simulink model "high_pass"  (R2024b)
settings: Solver=VariableStepAuto  StartTime=0.0  StopTime=10.0  RelTol=1e-3
libraries: dspsrcs4 x1
settings Model: Creator=woutlyen  LastModifiedBy=woutlyen

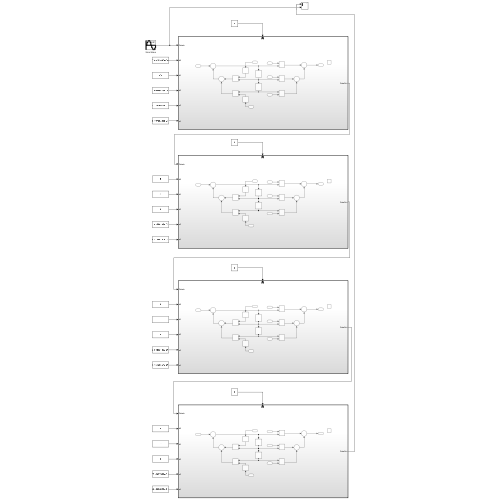
[thumbnail: Simulink's stored preview of the top-level diagram]
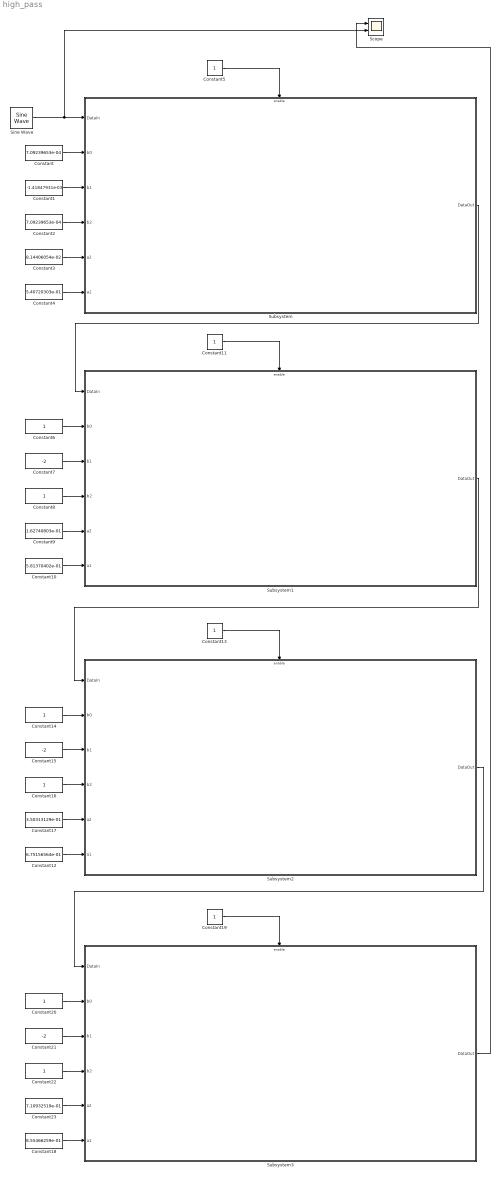
== system high_pass ==
  Constant : Constant  Value=7.09239653e-04  OutDataTypeStr=fixdt(1,27,23)
  Constant1 : Constant  Value=-1.41847931e-03  OutDataTypeStr=fixdt(1,27,23)
  Constant10 : Constant  Value=5.81370402e-01  OutDataTypeStr=fixdt(1,27,23)
  Constant{5,11,13,19} (4 alike) : Constant  OutDataTypeStr=boolean
  Constant12 : Constant  Value=6.75156564e-01  OutDataTypeStr=fixdt(1,27,23)
  Constant{6,8,14,16,20,22} (6 alike) : Constant  OutDataTypeStr=fixdt(1,27,23)
  Constant15 : Constant  Value=-2  OutDataTypeStr=fixdt(1,27,23)
  Constant17 : Constant  Value=3.50313129e-01  OutDataTypeStr=fixdt(1,27,23)
  Constant18 : Constant  Value=8.55466259e-01  OutDataTypeStr=fixdt(1,27,23)
  Constant2 : Constant  Value=7.09239653e-04  OutDataTypeStr=fixdt(1,27,23)
  Constant21 : Constant  Value=-2  OutDataTypeStr=fixdt(1,27,23)
  Constant23 : Constant  Value=7.10932519e-01  OutDataTypeStr=fixdt(1,27,23)
  Constant3 : Constant  Value=8.14406054e-02  OutDataTypeStr=fixdt(1,27,23)
  Constant4 : Constant  Value=5.40720303e-01  OutDataTypeStr=fixdt(1,27,23)
  Constant7 : Constant  Value=-2  OutDataTypeStr=fixdt(1,27,23)
  Constant9 : Constant  Value=1.62740803e-01  OutDataTypeStr=fixdt(1,27,23)
  Scope : Scope  NumInputPorts=2
  Sine Wave : dspsrcs4/Sine Wave  Amplitude=0.6  Frequency=16000  Phase=0  SampleMode=Discrete  OutComplex=Real  CompMethod=Table lookup  TableSize=Speed  SampleTime=1/48000  SamplesPerFrame=1  ResetState=Restart at time zero  OutputFrames=off  dataType=Fixed-point  wordLen=24  udDataType=sfix(16)  fracBitsMode=User-defined  numFracBits=23  OutDataTypeStr=fixdt(1,24,23)  LastOutDataTypeStr=fixdt(1,24,23)
  Subsystem : Subsystem
  Subsystem1 : Subsystem
  Subsystem2 : Subsystem
  Subsystem3 : Subsystem
  wires:
  Constant17/1 -> Subsystem2/5(a2)
  Constant19/1 -> Subsystem3/Enable
  Constant12/1 -> Subsystem2/6(a1)
  Subsystem1/1(DataOut) -> Subsystem2/1(DataIn)
  Constant5/1 -> Subsystem/Enable
  Constant20/1 -> Subsystem3/2(b0)
  Subsystem3/1(DataOut) -> Scope/1
  Constant4/1 -> Subsystem/6(a1)
  Constant18/1 -> Subsystem3/6(a1)
  Subsystem2/1(DataOut) -> Subsystem3/1(DataIn)
  Constant7/1 -> Subsystem1/3(b1)
  Constant13/1 -> Subsystem2/Enable
  Constant/1 -> Subsystem/2(b0)
  Constant22/1 -> Subsystem3/4(b2)
  Constant9/1 -> Subsystem1/5(a2)
  Constant11/1 -> Subsystem1/Enable
  Constant8/1 -> Subsystem1/4(b2)
  Constant1/1 -> Subsystem/3(b1)
  Constant6/1 -> Subsystem1/2(b0)
  Sine Wave/1 -> Scope/2, Subsystem/1(DataIn)
  Constant14/1 -> Subsystem2/2(b0)
  Constant3/1 -> Subsystem/5(a2)
  Constant2/1 -> Subsystem/4(b2)
  Constant10/1 -> Subsystem1/6(a1)
  Subsystem/1(DataOut) -> Subsystem1/1(DataIn)
  Constant15/1 -> Subsystem2/3(b1)
  Constant16/1 -> Subsystem2/4(b2)
  Constant23/1 -> Subsystem3/5(a2)
  Constant21/1 -> Subsystem3/3(b1)

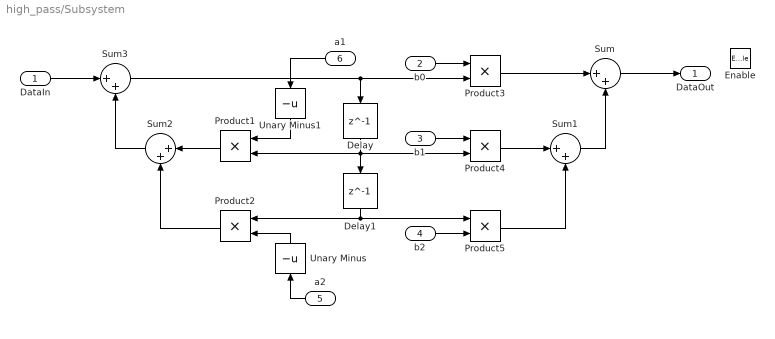
== system high_pass/Subsystem ==
  DataIn : Inport
  b0 : Inport  Port=2
  b1 : Inport  Port=3
  b2 : Inport  Port=4
  a2 : Inport  Port=5
  a1 : Inport  Port=6
  Enable : EnablePort
  Delay : Delay  DelayLength=1  InitialCondition=0
  Delay1 : Delay  DelayLength=1  InitialCondition=0
  Product{1..5} (5 alike) : Product  OutDataTypeStr=fixdt(1,27,23)
  Sum{,1..3} (4 alike) : Sum  Inputs=|++
  Unary Minus : UnaryMinus
  Unary Minus1 : UnaryMinus
  DataOut : Outport  VectorParamsAs1DForOutWhenUnconnected=off
  wires:
  Product4/1 -> Sum1/1
  b1/1 -> Product4/1
  Sum/1 -> DataOut/1
  Sum1/1 -> Sum/2
  b2/1 -> Product5/2
  a2/1 -> Unary Minus/1
  Delay1/1 -> Product2/1, Product5/1
  DataIn/1 -> Sum3/1
  Product2/1 -> Sum2/2
  Sum3/1 -> Delay/1, Product3/2
  Product1/1 -> Sum2/1
  Unary Minus1/1 -> Product1/1
  Sum2/1 -> Sum3/2
  Delay/1 -> Product4/2, Product1/2, Delay1/1
  Product3/1 -> Sum/1
  Unary Minus/1 -> Product2/2
  b0/1 -> Product3/1
  Product5/1 -> Sum1/2
  a1/1 -> Unary Minus1/1

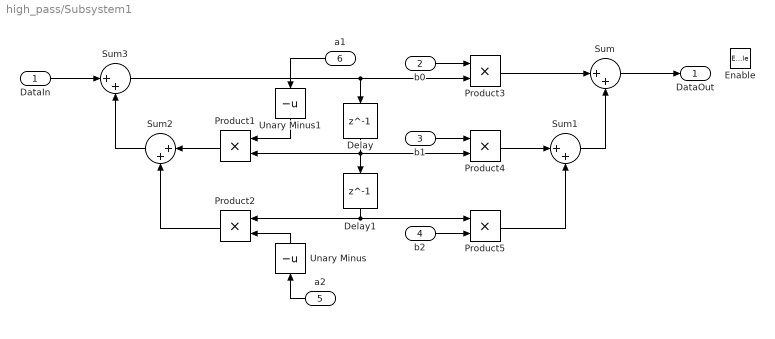
== system high_pass/Subsystem1 ==
  DataIn : Inport
  b0 : Inport  Port=2
  b1 : Inport  Port=3
  b2 : Inport  Port=4
  a2 : Inport  Port=5
  a1 : Inport  Port=6
  Enable : EnablePort
  Delay : Delay  DelayLength=1  InitialCondition=0
  Delay1 : Delay  DelayLength=1  InitialCondition=0
  Product{1..5} (5 alike) : Product  OutDataTypeStr=fixdt(1,27,23)
  Sum{,1..3} (4 alike) : Sum  Inputs=|++
  Unary Minus : UnaryMinus
  Unary Minus1 : UnaryMinus
  DataOut : Outport  VectorParamsAs1DForOutWhenUnconnected=off
  wires:
  Product4/1 -> Sum1/1
  b1/1 -> Product4/1
  Sum/1 -> DataOut/1
  Sum1/1 -> Sum/2
  b2/1 -> Product5/2
  a2/1 -> Unary Minus/1
  Delay1/1 -> Product2/1, Product5/1
  DataIn/1 -> Sum3/1
  Product2/1 -> Sum2/2
  Sum3/1 -> Delay/1, Product3/2
  Product1/1 -> Sum2/1
  Unary Minus1/1 -> Product1/1
  Sum2/1 -> Sum3/2
  Delay/1 -> Product4/2, Product1/2, Delay1/1
  Product3/1 -> Sum/1
  Unary Minus/1 -> Product2/2
  b0/1 -> Product3/1
  Product5/1 -> Sum1/2
  a1/1 -> Unary Minus1/1

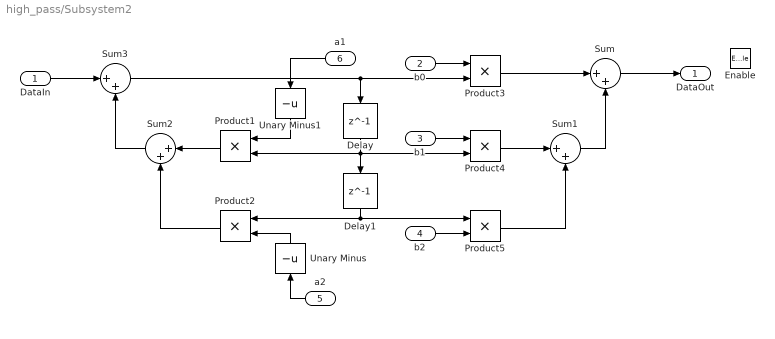
== system high_pass/Subsystem2 ==
  DataIn : Inport
  b0 : Inport  Port=2
  b1 : Inport  Port=3
  b2 : Inport  Port=4
  a2 : Inport  Port=5
  a1 : Inport  Port=6
  Enable : EnablePort
  Delay : Delay  DelayLength=1  InitialCondition=0
  Delay1 : Delay  DelayLength=1  InitialCondition=0
  Product{1..5} (5 alike) : Product  OutDataTypeStr=fixdt(1,27,23)
  Sum{,1..3} (4 alike) : Sum  Inputs=|++
  Unary Minus : UnaryMinus
  Unary Minus1 : UnaryMinus
  DataOut : Outport  VectorParamsAs1DForOutWhenUnconnected=off
  wires:
  Product4/1 -> Sum1/1
  b1/1 -> Product4/1
  Sum/1 -> DataOut/1
  Sum1/1 -> Sum/2
  b2/1 -> Product5/2
  a2/1 -> Unary Minus/1
  Delay1/1 -> Product2/1, Product5/1
  DataIn/1 -> Sum3/1
  Product2/1 -> Sum2/2
  Sum3/1 -> Delay/1, Product3/2
  Product1/1 -> Sum2/1
  Unary Minus1/1 -> Product1/1
  Sum2/1 -> Sum3/2
  Delay/1 -> Product4/2, Product1/2, Delay1/1
  Product3/1 -> Sum/1
  Unary Minus/1 -> Product2/2
  b0/1 -> Product3/1
  Product5/1 -> Sum1/2
  a1/1 -> Unary Minus1/1

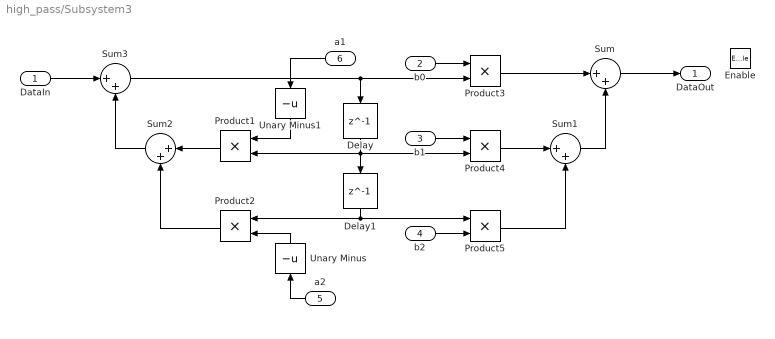
== system high_pass/Subsystem3 ==
  DataIn : Inport
  b0 : Inport  Port=2
  b1 : Inport  Port=3
  b2 : Inport  Port=4
  a2 : Inport  Port=5
  a1 : Inport  Port=6
  Enable : EnablePort
  Delay : Delay  DelayLength=1  InitialCondition=0
  Delay1 : Delay  DelayLength=1  InitialCondition=0
  Product{1..5} (5 alike) : Product  OutDataTypeStr=fixdt(1,27,23)
  Sum{,1..3} (4 alike) : Sum  Inputs=|++
  Unary Minus : UnaryMinus
  Unary Minus1 : UnaryMinus
  DataOut : Outport  VectorParamsAs1DForOutWhenUnconnected=off
  wires:
  Product4/1 -> Sum1/1
  b1/1 -> Product4/1
  Sum/1 -> DataOut/1
  Sum1/1 -> Sum/2
  b2/1 -> Product5/2
  a2/1 -> Unary Minus/1
  Delay1/1 -> Product2/1, Product5/1
  DataIn/1 -> Sum3/1
  Product2/1 -> Sum2/2
  Sum3/1 -> Delay/1, Product3/2
  Product1/1 -> Sum2/1
  Unary Minus1/1 -> Product1/1
  Sum2/1 -> Sum3/2
  Delay/1 -> Product4/2, Product1/2, Delay1/1
  Product3/1 -> Sum/1
  Unary Minus/1 -> Product2/2
  b0/1 -> Product3/1
  Product5/1 -> Sum1/2
  a1/1 -> Unary Minus1/1
